simulink model "modelRLC_TRANSFORMATA_szum"  (R2022a)
settings: Solver=ode4  StartTime=0.0  StopTime=T  FixedStep=1/Fs  RelTol=1e-3
values from neighbouring files (symbols this model uses):
  C = 10e-9    (= 1e-08)    [RLC_analysis.m]
  L = 10e-3    (= 0.01)    [RLC_analysis.m]
  R = 100    [RLC_analysis.m]
  seed = 0    [RLC_analysis.m]
  variance = 3    [RLC_analysis.m]
settings Model: Creator=domin  LastModifiedBy=domin

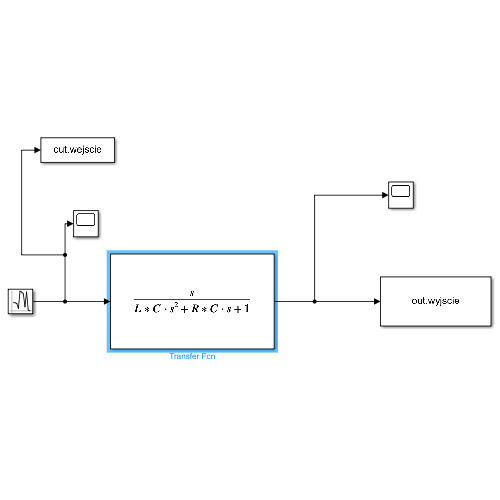
[thumbnail: Simulink's stored preview of the top-level diagram]
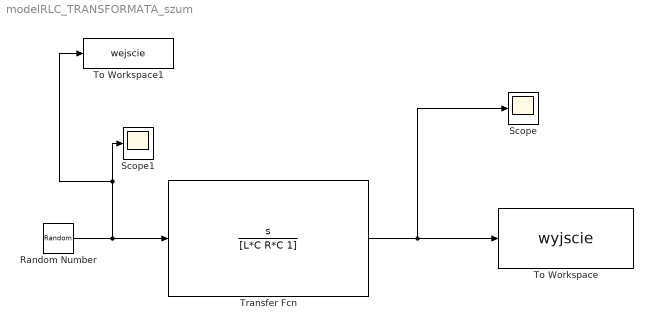
== system modelRLC_TRANSFORMATA_szum ==
  Random Number : RandomNumber  Mean=mean  Variance=variance  Seed=seed
  Scope : Scope
  Scope1 : Scope
  To Workspace : ToWorkspace  VariableName=wyjscie  SampleTime=-1
  To Workspace1 : ToWorkspace  VariableName=wejscie  SampleTime=-1
  Transfer Fcn : TransferFcn  Numerator=[1 0]  Denominator=[L*C R*C 1]
  wires:
  Random Number/1 -> Transfer Fcn/1, To Workspace1/1, Scope1/1
  Transfer Fcn/1 -> Scope/1, To Workspace/1
